simulink library "lib_Convection_HydraulicDiameter"  (R2015a)
settings: Solver=ode45  StartTime=0.0  StopTime=10.0  RelTol=1e-3
settings Model: Creator=jlkratz  LastModifiedBy=jlkratz

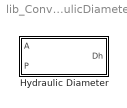
== system lib_Convection_HydraulicDiameter ==
  Hydraulic Diameter : Subsystem  mask(TSAT: Hydraulic Diameter){}
      mask help: This block calculates the hydraulic diameter (Dh) of an arbitrary shape based on its area (A) and perimeter (P). The units of the inputs must be consistent and the units of the outputs will be the same as the length unit used in the inputs. The hydrualic diameter is useful for evaluating heat transfer in non-circular tubes.
      mask Help: web(which('Convection_TSAT_HydraulicDiameter.html'),'-helpbrowser')

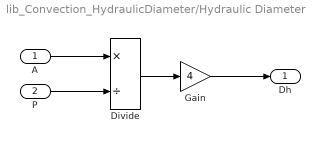
== system lib_Convection_HydraulicDiameter/Hydraulic Diameter ==
  A : Inport
  P : Inport  Port=2
  Divide : Product  Inputs=*/
  Gain : Gain  Gain=4
  Dh : Outport
  wires:
  Gain/1 -> Dh/1
  Divide/1 -> Gain/1
  P/1 -> Divide/2
  A/1 -> Divide/1
